simulink model "RefModel_FlightPerf"  (R2020b)
settings: Solver=ode1  StartTime=0.0  StopTime=10.0  FixedStep=SimParam.FightPerf.Ts_base  RelTol=1e-3
(part 1 of 2)
settings Model: Creator=sl  LastModifiedBy=sl
settings DataIOCC: SaveOutput=off  SaveTime=off
settings OptimizationCC: DefaultParameterBehavior=Inlined  EnhancedBackFolding=on  PassReuseOutputArgsAs=Individual arguments  ZeroExternalMemoryAtStartup=off  ZeroInternalMemoryAtStartup=off  OptimizeBlockOrder=speed  DifferentSizesBufferReuse=on  OptimizationCustomize=off  EfficientTunableParamExpr=on
settings DebuggingCC: InheritedTsInSrcMsg=none  ParameterPrecisionLossMsg=none  ParameterTunabilityLossMsg=error  UnconnectedInputMsg=none  UnconnectedOutputMsg=none  UnconnectedLineMsg=none  SFUnusedDataAndEventsDiag=none
settings HardwareCC: ProdBitPerPointer=32  ProdBitPerSizeT=32  ProdBitPerPtrDiffT=32  ProdLargestAtomicInteger=Long  ProdLargestAtomicFloat=Double  ProdWordSize=32  ProdHWDeviceType=ARM Compatible->ARM Cortex
settings ModelReferenceCC: ModelReferenceNumInstancesAllowed=Single  PropagateVarSize=During execution
settings SFSimCC: MATLABDynamicMemAlloc=off
settings RTWCC: Description=Embedded Coder  SystemTargetFile=ert.tlc  TemplateMakefile=ert_default_tmf  GenerateReport=on  IncludeHyperlinkInReport=on  LaunchReport=on  GenerateTraceInfo=on  GenerateTraceReport=on  GenerateTraceReportSl=on  GenerateTraceReportSf=on  GenerateTraceReportEml=on
settings CodeAppCC: ForceParamTrailComments=on  IgnoreCustomStorageClasses=off  MaxIdLength=48  OperatorAnnotations=on  SimulinkDataObjDesc=on  SFDataObjDesc=on  MATLABFcnDesc=on  InsertBlockDesc=on  StateflowObjectComments=on  MATLABSourceComments=on
settings ERTTargetCC: TargetLangStandard=C99 (ISO)  GenerateSampleERTMain=on  CombineOutputUpdateFcns=off  LogVarNameModifier=none  SupportVariableSizeSignals=on  InlinedParameterPlacement=NonHierarchical  ERTCustomFileTemplate=example_file_process.tlc

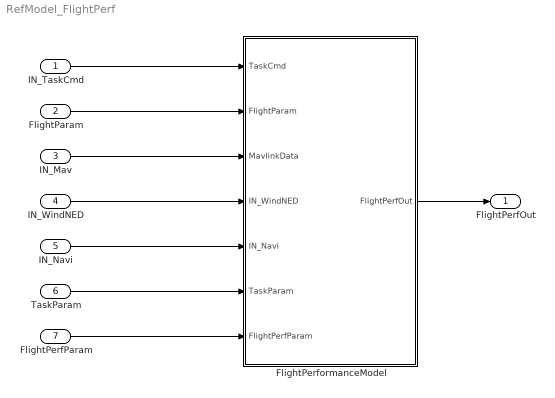
== system RefModel_FlightPerf ==
  IN_TaskCmd : Inport  OutDataTypeStr=Bus: BUS_TASK_PATH_OutParam  BusOutputAsStruct=on
  FlightParam : Inport  Port=2  OutDataTypeStr=Bus: BUS_TASK_COMMON_OutParam  BusOutputAsStruct=on
  IN_Mav : Inport  Port=3  OutDataTypeStr=Bus: BUS_MAVLINK_TO_FIRM  PortDimensions=1  BusOutputAsStruct=on
  IN_WindNED : Inport  Port=4  OutDataTypeStr=Bus: BUS_NAVI_GlobalWindEst
  IN_Navi : Inport  Port=5  OutDataTypeStr=Bus: BUS_NAVI_FilterOut
  TaskParam : Inport  Port=6  OutDataTypeStr=Bus: BUS_TASK_PARAM  BusOutputAsStruct=on
  FlightPerfParam : Inport  Port=7  OutDataTypeStr=Bus: BUS_FLIGHTPERF_PARAM  BusOutputAsStruct=on
  FlightPerformanceModel : Subsystem
  FlightPerfOut : Outport  OutDataTypeStr=Bus: BUS_FLIGHTPERF_OUT
  wires:
  IN_Mav/1 -> FlightPerformanceModel/3(MavlinkData)
  FlightPerformanceModel/1(FlightPerfOut) -> FlightPerfOut/1
  FlightParam/1 -> FlightPerformanceModel/2(FlightParam)
  IN_TaskCmd/1 -> FlightPerformanceModel/1(TaskCmd)
  IN_WindNED/1 -> FlightPerformanceModel/4(IN_WindNED)
  IN_Navi/1 -> FlightPerformanceModel/5(IN_Navi)
  TaskParam/1 -> FlightPerformanceModel/6(TaskParam)
  FlightPerfParam/1 -> FlightPerformanceModel/7(FlightPerfParam)

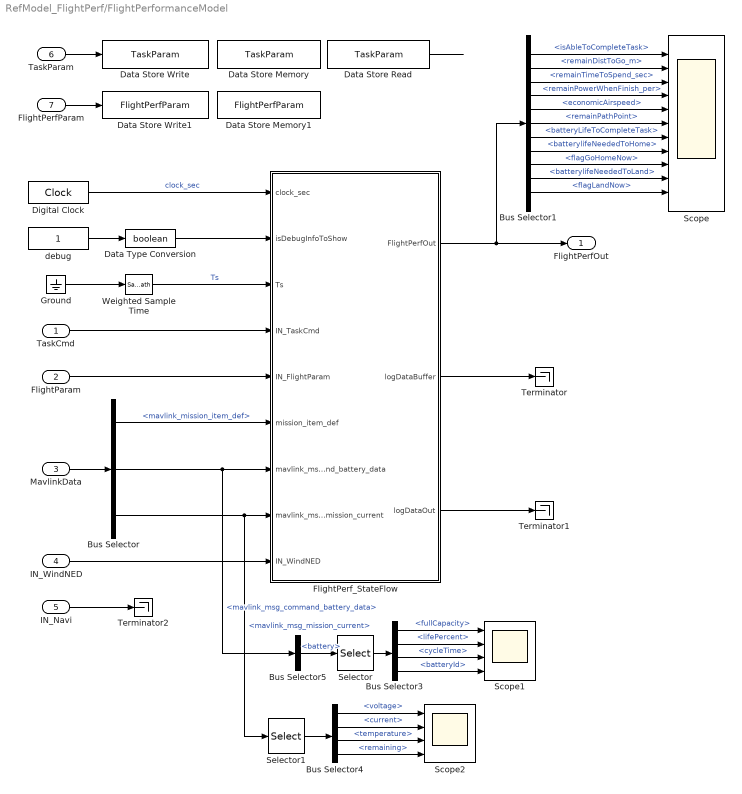
== system RefModel_FlightPerf/FlightPerformanceModel ==
  TaskCmd : Inport
  FlightParam : Inport  Port=2
  MavlinkData : Inport  Port=3
  IN_WindNED : Inport  Port=4
  IN_Navi : Inport  Port=5
  TaskParam : Inport  Port=6
  FlightPerfParam : Inport  Port=7
  Bus Selector : BusSelector  OutputSignals=mavlink_mission_item_def,mavlink_msg_command_battery_data,mavlink_msg_mission_current
  Bus Selector1 : BusSelector  OutputSignals=isAbleToCompleteTask,remainDistToGo_m,remainTimeToSpend_sec,remainPowerWhenFinish_per,economicAirspeed,remainPathPoint,batteryLifeToCompleteTask,batterylifeNeededToHome,flagGoHomeNow,batterylifeNeededToLand,flagLandNow
  Bus Selector3 : BusSelector  OutputSignals=fullCapacity,lifePercent,cycleTime,batteryId
  Bus Selector4 : BusSelector  OutputSignals=voltage,current,temperature,remaining
  Bus Selector5 : BusSelector  OutputSignals=battery
  Data Store Memory : DataStoreMemory  DataStoreName=TaskParam  ReadBeforeWriteMsg=warning  WriteAfterWriteMsg=warning  WriteAfterReadMsg=warning  ShowAdditionalParam=off  OutDataTypeStr=Bus: BUS_TASK_PARAM  Dimensions=1
  Data Store Memory1 : DataStoreMemory  DataStoreName=FlightPerfParam  ReadBeforeWriteMsg=warning  WriteAfterWriteMsg=warning  WriteAfterReadMsg=warning  ShowAdditionalParam=off  OutDataTypeStr=Bus: BUS_FLIGHTPERF_PARAM  Dimensions=1
  Data Store Read : DataStoreRead  DataStoreName=TaskParam
  Data Store Write : DataStoreWrite  DataStoreName=TaskParam
  Data Store Write1 : DataStoreWrite  DataStoreName=FlightPerfParam
  Data Type Conversion : DataTypeConversion  OutDataTypeStr=boolean
  Digital Clock : DigitalClock  SampleTime=-1
  FlightPerf_StateFlow : Stateflow chart  TreatAsAtomicUnit=on
  Ground : Ground
  Scope : Scope  NumInputPorts=11
  Scope1 : Scope  NumInputPorts=4
  Scope2 : Scope  NumInputPorts=4
  Selector : Selector  InputPortWidth=3  IndexOptions=Index vector (dialog)  Indices=1  OutputSizes=1
  Selector1 : Selector  InputPortWidth=TASK_PARAM_V1000.maxNumBattery  IndexOptions=Index vector (dialog)  Indices=1  OutputSizes=1
  Terminator : Terminator
  Terminator1 : Terminator
  Terminator2 : Terminator
  Weighted Sample Time : SampleTimeMath  TsampMathOp=Ts Only
  debug : Constant
  FlightPerfOut : Outport
  wires:
  FlightParam/1 -> FlightPerf_StateFlow/5(IN_FlightParam)
  debug/1 -> Data Type Conversion/1
  Data Type Conversion/1 -> FlightPerf_StateFlow/2(isDebugInfoToShow)
  Weighted Sample Time/1 -> FlightPerf_StateFlow/3(Ts)  "Ts"
  Digital Clock/1 -> FlightPerf_StateFlow/1(clock_sec)  "clock_sec"
  TaskCmd/1 -> FlightPerf_StateFlow/4(IN_TaskCmd)
  MavlinkData/1 -> Bus Selector/1
  Ground/1 -> Weighted Sample Time/1
  Bus Selector/1 -> FlightPerf_StateFlow/6(mission_item_def)  "<mavlink_mission_item_def>"
  Bus Selector/2 -> Bus Selector5/1, FlightPerf_StateFlow/7(mavlink_msg_command_battery_data)  "<mavlink_msg_command_battery_data>"
  FlightPerf_StateFlow/1(FlightPerfOut) -> Bus Selector1/1, FlightPerfOut/1
  Bus Selector/3 -> Selector1/1, FlightPerf_StateFlow/8(mavlink_msg_mission_current)  "<mavlink_msg_mission_current>"
  IN_WindNED/1 -> FlightPerf_StateFlow/9(IN_WindNED)
  Bus Selector1/1 -> Scope/1  "<isAbleToCompleteTask>"
  Bus Selector1/2 -> Scope/2  "<remainDistToGo_m>"
  Bus Selector1/3 -> Scope/3  "<remainTimeToSpend_sec>"
  Bus Selector1/4 -> Scope/4  "<remainPowerWhenFinish_per>"
  Bus Selector1/5 -> Scope/5  "<economicAirspeed>"
  Bus Selector1/6 -> Scope/6  "<remainPathPoint>"
  Bus Selector1/7 -> Scope/7  "<batteryLifeToCompleteTask>"
  Bus Selector1/8 -> Scope/8  "<batterylifeNeededToHome>"
  Bus Selector1/9 -> Scope/9  "<flagGoHomeNow>"
  Bus Selector1/10 -> Scope/10  "<batterylifeNeededToLand>"
  IN_Navi/1 -> Terminator2/1
  Bus Selector3/1 -> Scope1/1  "<fullCapacity>"
  Bus Selector3/2 -> Scope1/2  "<lifePercent>"
  Bus Selector3/3 -> Scope1/3  "<cycleTime>"
  Bus Selector3/4 -> Scope1/4  "<batteryId>"
  Bus Selector4/1 -> Scope2/1  "<voltage>"
  Bus Selector4/2 -> Scope2/2  "<current>"
  Bus Selector4/3 -> Scope2/3  "<temperature>"
  Bus Selector4/4 -> Scope2/4  "<remaining>"
  Selector/1 -> Bus Selector3/1
  Selector1/1 -> Bus Selector4/1
  Bus Selector5/1 -> Selector/1  "<battery>"
  TaskParam/1 -> Data Store Write/1
  FlightPerfParam/1 -> Data Store Write1/1
  Data Store Read/1 -> ?
  Bus Selector1/11 -> Scope/11  "<flagLandNow>"
  FlightPerf_StateFlow/2(logDataBuffer) -> Terminator/1
  FlightPerf_StateFlow/3(logDataOut) -> Terminator1/1
